simulink model "RL_Controller_sim"  (R2021a)
settings: Solver=VariableStepAuto  StartTime=0.0  StopTime=0.1  RelTol=1e-3
values from neighbouring files (symbols this model uses):
  fo = 50    [PI_Controller.m]    (also in RL_Controller_train.m)
  Iref = 2*Pref/Vg    [PI_Controller.m]    (also in RL_Controller_train.m)
  L = 15e-3    (= 0.015)    [PI_Controller.m]    (also in RL_Controller_train.m)
  R = 1e-3    (= 0.001)    [PI_Controller.m]    (also in RL_Controller_train.m)
  Ts = 1/fs    (= 2.5e-05)    [PI_Controller.m]    (also in RL_Controller_train.m)
  Tstep = Ts/500    (= 5e-08)    [RL_Controller_train.m]
  Vdc = 400    [PI_Controller.m]    (also in RL_Controller_train.m)
  Vg = 240*sqrt(2)    [PI_Controller.m]    (also in RL_Controller_train.m)
libraries: spsIGBTDiodeLib x4, spsVoltageMeasurementLib x2, spsDCVoltageSourceLib x1, spsSeriesRLCBranchLib x1, spsACVoltageSourceLib x1, spsGroundLib x1, spsCurrentMeasurementLib x1, rllib x1, spspowerguiLib x1
settings Model: Creator=ASUS-PC  LastModifiedBy=ASUS-PC
settings SolverCC: AlgebraicLoopSolver=TrustRegion
settings DebuggingCC: SFMachineParentedDataDiag=warning

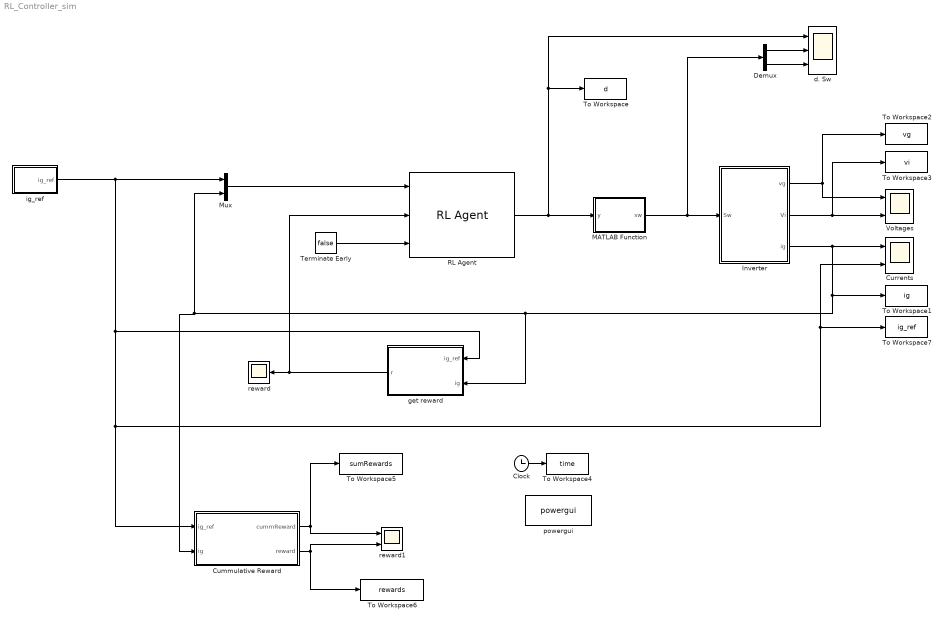
== system RL_Controller_sim ==
  Clock : Clock
  Cummulative Reward : MATLAB Function  TreatAsAtomicUnit=on  SystemSampleTime=Ts
  Currents : Scope  NumInputPorts=2
  Demux : Demux  Outputs=2
  Inverter : Subsystem
  MATLAB Function : MATLAB Function  TreatAsAtomicUnit=on  SystemSampleTime=Ts
  Mux : Mux  Inputs=2
  RL Agent : rllib/RL Agent  Agent=agent  ExternalActionAsInput=off  ProvideCumRwd=off  TreatAsDirectFeedthrough=on
  Terminate Early : Constant  Value=false
  To Workspace : ToWorkspace  VariableName=d  SampleTime=Ts
  To Workspace1 : ToWorkspace  VariableName=ig  SampleTime=Ts
  To Workspace2 : ToWorkspace  VariableName=vg  SampleTime=Ts
  To Workspace3 : ToWorkspace  VariableName=vi  SampleTime=Ts
  To Workspace4 : ToWorkspace  VariableName=time  SampleTime=Ts
  To Workspace5 : ToWorkspace  VariableName=sumRewards  SampleTime=Ts
  To Workspace6 : ToWorkspace  VariableName=rewards  SampleTime=Ts
  To Workspace7 : ToWorkspace  VariableName=ig_ref  SampleTime=Ts
  Voltages : Scope  NumInputPorts=2
  d. Sw : Scope  NumInputPorts=3
  get reward : Subsystem
  ig_ref : Subsystem
  powergui : spspowerguiLib/powergui  SimulationMode=Continuous  SampleTime=Tstep  frequency=60  Iterations=50  frequencyindice=0  Pbase=100e6  ErrMax=1e-4  UnitsV=kV  UnitsW=MW  buscounter=0  FunctionMessages=off  echomessages=off  EnableUseOfTLC=off  CurrentSourceSwitches=off  DisableSnubberDevices=off  DisableRonSwitches=off  DisableVfSwitches=off  DisplayEquations=off  AutomaticDiscreteSolvers=off  SolverType=Tustin/Backward Euler (TBE)  Interpol=off  ExternalGateDelay=off  methode=off  Ts=0  x0status=blocks  SPID=off  SwTol=0  HookPort=off  NonlinearTolerance=1e-4  nMaxIteration=100  ContinueOnMaxIteration=off  RestoreLinks=warning  ResistiveCurrentMeasurement=off  Frange=[0:2:500]  Ylog=off  Xlog=on  ShowGrid=off  save=off  variable=ZData  structure=Currents  ZoomFFT=off  StartTime=0.0  cycles=2  DisplayStyle=4  fundamental=50  FreqAxis=off  MaxFrequency=2500  frequencyindicesteady=1  RmsSteady=1  display=off
  reward : Scope
  reward1 : Scope  NumInputPorts=2
  wires:
  get reward/1(r) -> RL Agent/2, reward/1
  MATLAB Function/1(sw) -> Demux/1, Inverter/1(Sw)
  Inverter/1(vg) -> Voltages/1, To Workspace2/1
  Inverter/2(Vi) -> Voltages/2, To Workspace3/1
  Clock/1 -> To Workspace4/1
  RL Agent/1 -> MATLAB Function/1(y), To Workspace/1, d. Sw/1
  Terminate Early/1 -> RL Agent/3
  Demux/1 -> d. Sw/2
  Demux/2 -> d. Sw/3
  Mux/1 -> RL Agent/1
  Cummulative Reward/2(reward) -> reward1/2, To Workspace6/1
  ig_ref/1(ig_ref) -> get reward/1(ig_ref), Cummulative Reward/1(ig_ref), Currents/2, To Workspace7/1, Mux/1
  Inverter/3(ig) -> Currents/1, Mux/2, Cummulative Reward/2(ig), get reward/2(ig), To Workspace1/1
  Cummulative Reward/1(cummReward) -> reward1/1, To Workspace5/1

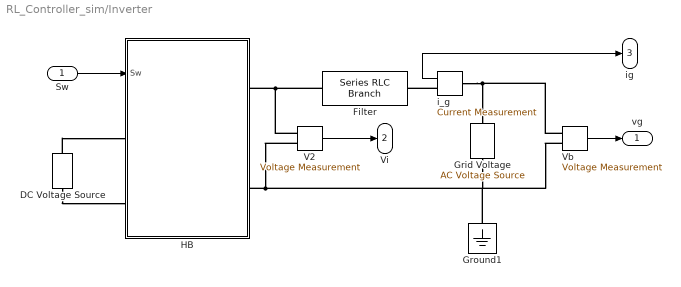
== system RL_Controller_sim/Inverter ==
  Sw : Inport
  DC Voltage Source : spsDCVoltageSourceLib/DC Voltage Source  Amplitude=Vdc  Measurements=None
  Filter : spsSeriesRLCBranchLib/Series RLC Branch  LConnTagsString=__new0  RConnTagsString=__new0  BranchType=RL  Resistance=R  Inductance=L  SetiL0=on  InitialCurrent=0  Capacitance=1e-6  Setx0=off  InitialVoltage=0  Measurements=Branch current
  Grid Voltage : spsACVoltageSourceLib/AC Voltage Source  Amplitude=Vg  Phase=0  Frequency=fo  SampleTime=0  Measurements=None  BusType=swing  Pref=10e3  Qref=0  Qmin=-inf  Qmax=+inf
  Ground1 : spsGroundLib/Ground  LConnTagsString=a
  HB : Subsystem
  V2 : spsVoltageMeasurementLib/Voltage Measurement  Tag=PoWeRsYsTeMmEaSuReMeNt  PhasorSimulation=off  OutputType=Magnitude  PSBequivalent=0
  Vb : spsVoltageMeasurementLib/Voltage Measurement  Tag=PoWeRsYsTeMmEaSuReMeNt  PhasorSimulation=off  OutputType=Magnitude  PSBequivalent=0
  i_g : spsCurrentMeasurementLib/Current Measurement  PhasorSimulation=off  OutputType=Complex  PSBequivalent=0
  vg : Outport  VectorParamsAs1DForOutWhenUnconnected=off
  Vi : Outport  Port=2  VectorParamsAs1DForOutWhenUnconnected=off
  ig : Outport  Port=3  VectorParamsAs1DForOutWhenUnconnected=off
  wires:
  Vb/1 -> vg/1
  Sw/1 -> HB/1(Sw)
  V2/1 -> Vi/1
  i_g/1 -> ig/1
  connections:
  DC Voltage Source/RConn1 -- HB/LConn1
  Vb/LConn1 -- Grid Voltage/RConn1 -- i_g/LConn1
  V2/LConn1 -- Filter/LConn1 -- HB/RConn1
  V2/LConn2 -- Grid Voltage/LConn1 -- Vb/LConn2 -- Ground1/LConn1 -- HB/RConn2
  DC Voltage Source/LConn1 -- HB/LConn2
  i_g/RConn1 -- Filter/RConn1

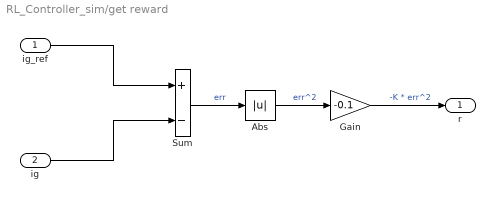
== system RL_Controller_sim/get reward ==
  ig_ref : Inport
  ig : Inport  Port=2
  Abs : Abs
  Gain : Gain  Gain=-0.1
  Sum : Sum  Inputs=+-
  r : Outport
  wires:
  ig_ref/1 -> Sum/1
  ig/1 -> Sum/2
  Abs/1 -> Gain/1  "err^2"
  Sum/1 -> Abs/1  "err"
  Gain/1 -> r/1  "-K * err^2"

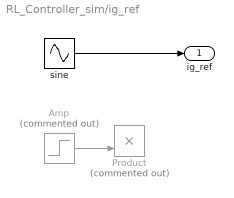
== system RL_Controller_sim/ig_ref ==
  Amp : Step  Commented=on  Time=0.055  Before=Iref  After=-Iref  SampleTime=0
  Product : Product  Commented=on
  sine : Sin  Amplitude=Iref  Frequency=2*pi*fo  SampleTime=0
  ig_ref : Outport  VectorParamsAs1DForOutWhenUnconnected=off
  wires:
  Amp/1 -> Product/2
  sine/1 -> ig_ref/1

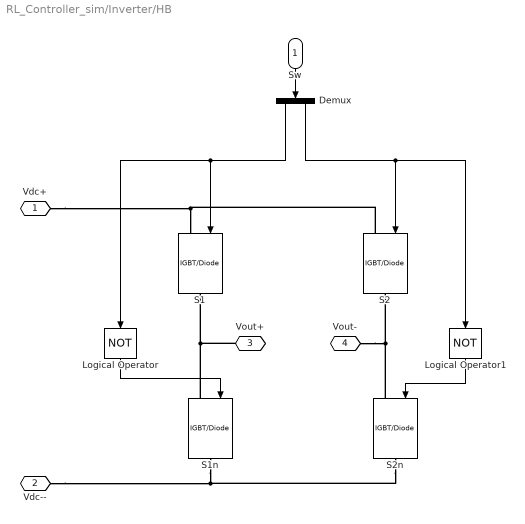
== system RL_Controller_sim/Inverter/HB ==
  Sw : Inport
  Demux : Demux  Outputs=2
  Logical Operator : Logic  Operator=NOT  AllPortsSameDT=off  OutDataTypeStr=boolean
  Logical Operator1 : Logic  Operator=NOT  AllPortsSameDT=off  OutDataTypeStr=boolean
  S1 : spsIGBTDiodeLib/IGBT//Diode  Ron=1e-3  Rs=1e5  Cs=inf  Measurements=off
  S1n : spsIGBTDiodeLib/IGBT//Diode  Ron=1e-3  Rs=1e5  Cs=inf  Measurements=off
  S2 : spsIGBTDiodeLib/IGBT//Diode  Ron=1e-3  Rs=1e5  Cs=inf  Measurements=off
  S2n : spsIGBTDiodeLib/IGBT//Diode  Ron=1e-3  Rs=1e5  Cs=inf  Measurements=off
  Vdc+ : PMIOPort  Side=Left
  Vdc-- : PMIOPort  Port=2  Side=Left
  Vout+ : PMIOPort  Port=3  Side=Right
  Vout- : PMIOPort  Port=4  Side=Right
  wires:
  Logical Operator/1 -> S1n/1
  Sw/1 -> Demux/1
  Demux/1 -> Logical Operator/1, S1/1
  Logical Operator1/1 -> S2n/1
  Demux/2 -> Logical Operator1/1, S2/1
  connections:
  S1n/RConn1 -- Vdc--/RConn1 -- S2n/RConn1
  S1n/LConn1 -- Vout+/RConn1 -- S1/RConn1
  S2n/LConn1 -- Vout-/RConn1 -- S2/RConn1
  S2/LConn1 -- Vdc+/RConn1 -- S1/LConn1

== matlab function RL_Controller_sim/MATLAB Function ==
  data: y input; sw output
function sw = fcn(y)
    sw = [-1 -1]';
    switch y
        case 0
            sw = [0 0]';
        case 1
            sw = [0 1]';
        case 2
            sw = [1 0]';
        case 3
            sw = [1 1]';
    end
end

== matlab function RL_Controller_sim/Cummulative Reward ==
  data: ig_ref input; cummReward output; ig input; reward output
function [cummReward, reward]= calcReward(ig_ref, ig)

    persistent sumReward;
    if isempty(sumReward)
        sumReward = 0;
    end
    
    % reward on this time step
    reward = abs(ig_ref-ig)*-0.1;
    
    % cummulative reward
    sumReward = sumReward+reward;
    
    % output to view on scope
    cummReward = sumReward;
end
